simulink model "fuzzyPD_Quadrotor"  (R2025a)
settings: Solver=VariableStepAuto  StartTime=0.0  StopTime=50  RelTol=1e-3
libraries: fuzblock x6, slpidlib x3, uavutilslib x1
settings Model: SimulationMode=accelerator  Creator=vinh1  LastModifiedBy=vinh1
settings RTWCC: Toolchain=MinGW64 | gmake (64-bit Windows)

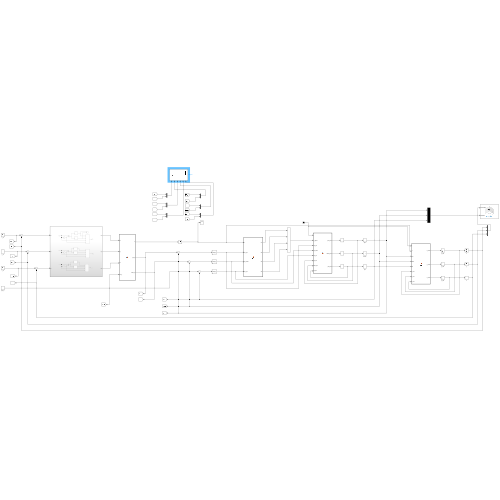
[thumbnail: Simulink's stored preview of the top-level diagram]
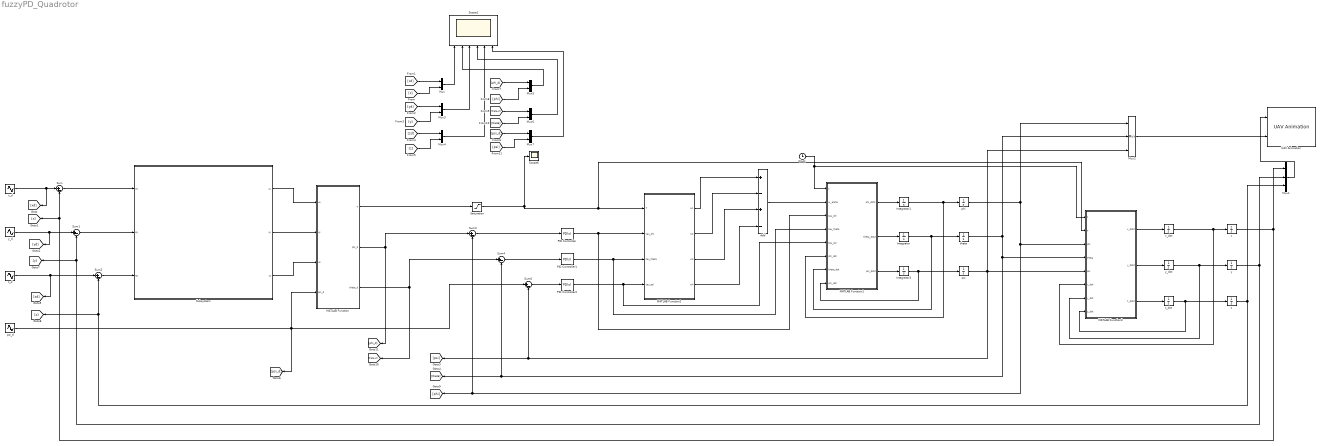
== system fuzzyPD_Quadrotor ==
  Add : Sum  Inputs=+-+-
  Clock : Clock
      settings: Decimation=200
  Integrator : Integrator
  Integrator1 : Integrator
  Integrator3 : Integrator
  MATLAB Function : MATLAB Function  TreatAsAtomicUnit=on
  MATLAB Function1 : MATLAB Function  TreatAsAtomicUnit=on
  MATLAB Function2 : MATLAB Function  TreatAsAtomicUnit=on
  MATLAB Function3 : MATLAB Function  TreatAsAtomicUnit=on
  Mux{,3..7} (6 alike) : Mux  Inputs=2
  Mux1 : Mux  Inputs=3
  Mux2 : Mux  Inputs=3
  PID Controller : slpidlib/PID Controller  Controller=PD  Form=Parallel  TimeDomain=Continuous-time  UseExternalTs=off  SampleTime=-1  IntegratorMethod=Forward Euler  FilterMethod=Forward Euler  ControllerParametersSource=internal  P=0.1  I=1  UseKiTs=off  D=1/3  UseExternalDerivativeSource=off  N=100  UseFilter=on  TunerSelectOption=Transfer Function Based (PID Tuner App)  InitialConditionSource=internal  InitialConditionForIntegrator=0  InitialConditionForFilter=0  DifferentiatorICPrevScaledInput=0  ExternalReset=none  TrackingMode=off  Kt=1  LimitOutput=off  SatLimitsSource=internal  UpperSaturationLimit=inf  LowerSaturationLimit=-inf  LinearizeAsGain=on  AntiWindupMode=none  Kb=1  LimitIntegrator=off  UpperIntegratorSaturationLimit=inf  LowerIntegratorSaturationLimit=-inf  POutMin=[]  POutMax=[]  IOutMin=[]  IOutMax=[]  DOutMin=[]  DOutMax=[]  NOutMin=[]  NOutMax=[]  SumOutMin=[]  SumOutMax=[]  SaturationOutMin=[]  SaturationOutMax=[]  PParamMin=[]  PParamMax=[]  IParamMin=[]  IParamMax=[]  DParamMin=[]  DParamMax=[]  NParamMin=[]  NParamMax=[]  KbParamMin=[]  KbParamMax=[]  KtParamMin=[]  KtParamMax=[]  KbOutMin=[]  KbOutMax=[]  KtOutMin=[]  KtOutMax=[]  IntegratorOutMin=[]  IntegratorOutMax=[]  FilterOutMin=[]  FilterOutMax=[]  SumI1OutMin=[]  SumI1OutMax=[]  SumI2OutMin=[]  SumI2OutMax=[]  SumI3OutMin=[]  SumI3OutMax=[]  SumI4OutMin=[]  SumI4OutMax=[]  SumDOutMin=[]  SumDOutMax=[]  DifferentiatorOutMin=[]  DifferentiatorOutMax=[]  FilterDiffOutCoefMin=[]  FilterDiffOutCoefMax=[]  ReciprocalOutMin=[]  ReciprocalOutMax=[]  SumDenOutMin=[]  SumDenOutMax=[]  SumNumOutMin=[]  SumNumOutMax=[]  DivideOutMin=[]  DivideOutMax=[]  UdiffTsProdOutMin=[]  UdiffTsProdOutMax=[]  NTsProdOutMin=[]  NTsProdOutMax=[]  UintegralTsProdOutMin=[]  UintegralTsProdOutMax=[]  UngainTsProdOutMin=[]  UngainTsProdOutMax=[]  ClampingZeroOutDataTypeStr=Inherit: Inherit via back propagation  ClampingZeroOutMin=[]  ClampingZeroOutMax=[]  FilterDenConstantOutDataTypeStr=Inherit: Inherit via back propagation  FilterDenConstantOutMin=[]  FilterDenConstantOutMax=[]  PCopyOutDataTypeStr=Inherit: Inherit via back propagation  PCopyOutMin=[]  PCopyOutMax=[]  NCopyOutDataTypeStr=Inherit: Inherit via back propagation  NCopyOutMin=[]  NCopyOutMax=[]  IntegratorContinuousStateAttributes=''  IntegratorStateMustResolveToSignalObject=off  IntegratorRTWStateStorageClass=Auto  FilterContinuousStateAttributes=''  FilterStateMustResolveToSignalObject=off  FilterRTWStateStorageClass=Auto  ParallelPVariant=InternalParameters  IdealPVariant=Disabled  IVariant=Disabled  DVariant=InternalParameters  IntegratorVariant=Disabled  SatVariant=Disabled  AWVariant=Disabled  PCopyVariant=Disabled  TRVariant=Disabled  FdbkBlocksVariant=Forward  IdealPFdbkVariant=Disabled  SatFdbkVariant=Disabled  DerivativeFilterVariant=ContFilter  NVariant=InternalParameters  NCopyVariant=Disabled  FilterICVariant=InternalICsFilter  IntegratorICVariant=Disabled  ExternalResetVariant=Disabled  TRSumVariant=Passthrough  SumFdbkVariant=Disabled  SumVariant=Sum_PD  TsampFilterVariant=InternalTs  TsampNgainVariant=Passthrough  TsampIntegralVariant=Disabled_SignalSpec  ExternalSaturationOutDataTypeStr=Inherit: Same as second input  DerivativeSourceVariant=ErrorSignal  PreIntVariant=InternalPreInt
  PID Controller1 : slpidlib/PID Controller  Controller=PD  Form=Parallel  TimeDomain=Continuous-time  UseExternalTs=off  SampleTime=-1  IntegratorMethod=Forward Euler  FilterMethod=Forward Euler  ControllerParametersSource=internal  P=0.1  I=1  UseKiTs=off  D=1/3  UseExternalDerivativeSource=off  N=100  UseFilter=on  TunerSelectOption=Transfer Function Based (PID Tuner App)  InitialConditionSource=internal  InitialConditionForIntegrator=0  InitialConditionForFilter=0  DifferentiatorICPrevScaledInput=0  ExternalReset=none  TrackingMode=off  Kt=1  LimitOutput=off  SatLimitsSource=internal  UpperSaturationLimit=inf  LowerSaturationLimit=-inf  LinearizeAsGain=on  AntiWindupMode=none  Kb=1  LimitIntegrator=off  UpperIntegratorSaturationLimit=inf  LowerIntegratorSaturationLimit=-inf  POutMin=[]  POutMax=[]  IOutMin=[]  IOutMax=[]  DOutMin=[]  DOutMax=[]  NOutMin=[]  NOutMax=[]  SumOutMin=[]  SumOutMax=[]  SaturationOutMin=[]  SaturationOutMax=[]  PParamMin=[]  PParamMax=[]  IParamMin=[]  IParamMax=[]  DParamMin=[]  DParamMax=[]  NParamMin=[]  NParamMax=[]  KbParamMin=[]  KbParamMax=[]  KtParamMin=[]  KtParamMax=[]  KbOutMin=[]  KbOutMax=[]  KtOutMin=[]  KtOutMax=[]  IntegratorOutMin=[]  IntegratorOutMax=[]  FilterOutMin=[]  FilterOutMax=[]  SumI1OutMin=[]  SumI1OutMax=[]  SumI2OutMin=[]  SumI2OutMax=[]  SumI3OutMin=[]  SumI3OutMax=[]  SumI4OutMin=[]  SumI4OutMax=[]  SumDOutMin=[]  SumDOutMax=[]  DifferentiatorOutMin=[]  DifferentiatorOutMax=[]  FilterDiffOutCoefMin=[]  FilterDiffOutCoefMax=[]  ReciprocalOutMin=[]  ReciprocalOutMax=[]  SumDenOutMin=[]  SumDenOutMax=[]  SumNumOutMin=[]  SumNumOutMax=[]  DivideOutMin=[]  DivideOutMax=[]  UdiffTsProdOutMin=[]  UdiffTsProdOutMax=[]  NTsProdOutMin=[]  NTsProdOutMax=[]  UintegralTsProdOutMin=[]  UintegralTsProdOutMax=[]  UngainTsProdOutMin=[]  UngainTsProdOutMax=[]  ClampingZeroOutDataTypeStr=Inherit: Inherit via back propagation  ClampingZeroOutMin=[]  ClampingZeroOutMax=[]  FilterDenConstantOutDataTypeStr=Inherit: Inherit via back propagation  FilterDenConstantOutMin=[]  FilterDenConstantOutMax=[]  PCopyOutDataTypeStr=Inherit: Inherit via back propagation  PCopyOutMin=[]  PCopyOutMax=[]  NCopyOutDataTypeStr=Inherit: Inherit via back propagation  NCopyOutMin=[]  NCopyOutMax=[]  IntegratorContinuousStateAttributes=''  IntegratorStateMustResolveToSignalObject=off  IntegratorRTWStateStorageClass=Auto  FilterContinuousStateAttributes=''  FilterStateMustResolveToSignalObject=off  FilterRTWStateStorageClass=Auto  ParallelPVariant=InternalParameters  IdealPVariant=Disabled  IVariant=Disabled  DVariant=InternalParameters  IntegratorVariant=Disabled  SatVariant=Disabled  AWVariant=Disabled  PCopyVariant=Disabled  TRVariant=Disabled  FdbkBlocksVariant=Forward  IdealPFdbkVariant=Disabled  SatFdbkVariant=Disabled  DerivativeFilterVariant=ContFilter  NVariant=InternalParameters  NCopyVariant=Disabled  FilterICVariant=InternalICsFilter  IntegratorICVariant=Disabled  ExternalResetVariant=Disabled  TRSumVariant=Passthrough  SumFdbkVariant=Disabled  SumVariant=Sum_PD  TsampFilterVariant=InternalTs  TsampNgainVariant=Passthrough  TsampIntegralVariant=Disabled_SignalSpec  ExternalSaturationOutDataTypeStr=Inherit: Same as second input  DerivativeSourceVariant=ErrorSignal  PreIntVariant=InternalPreInt
  PID Controller2 : slpidlib/PID Controller  Controller=PD  Form=Parallel  TimeDomain=Continuous-time  UseExternalTs=off  SampleTime=-1  IntegratorMethod=Forward Euler  FilterMethod=Forward Euler  ControllerParametersSource=internal  P=0.1  I=1  UseKiTs=off  D=1/3  UseExternalDerivativeSource=off  N=100  UseFilter=on  TunerSelectOption=Transfer Function Based (PID Tuner App)  InitialConditionSource=internal  InitialConditionForIntegrator=0  InitialConditionForFilter=0  DifferentiatorICPrevScaledInput=0  ExternalReset=none  TrackingMode=off  Kt=1  LimitOutput=off  SatLimitsSource=internal  UpperSaturationLimit=inf  LowerSaturationLimit=-inf  LinearizeAsGain=on  AntiWindupMode=none  Kb=1  LimitIntegrator=off  UpperIntegratorSaturationLimit=inf  LowerIntegratorSaturationLimit=-inf  POutMin=[]  POutMax=[]  IOutMin=[]  IOutMax=[]  DOutMin=[]  DOutMax=[]  NOutMin=[]  NOutMax=[]  SumOutMin=[]  SumOutMax=[]  SaturationOutMin=[]  SaturationOutMax=[]  PParamMin=[]  PParamMax=[]  IParamMin=[]  IParamMax=[]  DParamMin=[]  DParamMax=[]  NParamMin=[]  NParamMax=[]  KbParamMin=[]  KbParamMax=[]  KtParamMin=[]  KtParamMax=[]  KbOutMin=[]  KbOutMax=[]  KtOutMin=[]  KtOutMax=[]  IntegratorOutMin=[]  IntegratorOutMax=[]  FilterOutMin=[]  FilterOutMax=[]  SumI1OutMin=[]  SumI1OutMax=[]  SumI2OutMin=[]  SumI2OutMax=[]  SumI3OutMin=[]  SumI3OutMax=[]  SumI4OutMin=[]  SumI4OutMax=[]  SumDOutMin=[]  SumDOutMax=[]  DifferentiatorOutMin=[]  DifferentiatorOutMax=[]  FilterDiffOutCoefMin=[]  FilterDiffOutCoefMax=[]  ReciprocalOutMin=[]  ReciprocalOutMax=[]  SumDenOutMin=[]  SumDenOutMax=[]  SumNumOutMin=[]  SumNumOutMax=[]  DivideOutMin=[]  DivideOutMax=[]  UdiffTsProdOutMin=[]  UdiffTsProdOutMax=[]  NTsProdOutMin=[]  NTsProdOutMax=[]  UintegralTsProdOutMin=[]  UintegralTsProdOutMax=[]  UngainTsProdOutMin=[]  UngainTsProdOutMax=[]  ClampingZeroOutDataTypeStr=Inherit: Inherit via back propagation  ClampingZeroOutMin=[]  ClampingZeroOutMax=[]  FilterDenConstantOutDataTypeStr=Inherit: Inherit via back propagation  FilterDenConstantOutMin=[]  FilterDenConstantOutMax=[]  PCopyOutDataTypeStr=Inherit: Inherit via back propagation  PCopyOutMin=[]  PCopyOutMax=[]  NCopyOutDataTypeStr=Inherit: Inherit via back propagation  NCopyOutMin=[]  NCopyOutMax=[]  IntegratorContinuousStateAttributes=''  IntegratorStateMustResolveToSignalObject=off  IntegratorRTWStateStorageClass=Auto  FilterContinuousStateAttributes=''  FilterStateMustResolveToSignalObject=off  FilterRTWStateStorageClass=Auto  ParallelPVariant=InternalParameters  IdealPVariant=Disabled  IVariant=Disabled  DVariant=InternalParameters  IntegratorVariant=Disabled  SatVariant=Disabled  AWVariant=Disabled  PCopyVariant=Disabled  TRVariant=Disabled  FdbkBlocksVariant=Forward  IdealPFdbkVariant=Disabled  SatFdbkVariant=Disabled  DerivativeFilterVariant=ContFilter  NVariant=InternalParameters  NCopyVariant=Disabled  FilterICVariant=InternalICsFilter  IntegratorICVariant=Disabled  ExternalResetVariant=Disabled  TRSumVariant=Passthrough  SumFdbkVariant=Disabled  SumVariant=Sum_PD  TsampFilterVariant=InternalTs  TsampNgainVariant=Passthrough  TsampIntegralVariant=Disabled_SignalSpec  ExternalSaturationOutDataTypeStr=Inherit: Same as second input  DerivativeSourceVariant=ErrorSignal  PreIntVariant=InternalPreInt
  Saturation : Saturate  UpperLimit=130  LowerLimit=0
  Scope1 : Scope  NumInputPorts=6
      settings: ActiveDisplayYMinimum=-0.63879250975812629  ActiveDisplayYMaximum=0.70191029435128827
  Scope6 : Scope
      settings: ActiveDisplayYMinimum=9.3887609139201285  ActiveDisplayYMaximum=11.61040929343401  DataLoggingVariableName=ScopeData6
  Subsystem : Subsystem
  Sum{,1..4,6} (6 alike) : Sum  Inputs=|+-
  UAV Animation : uavutilslib/UAV Animation  NumUAV=1  DynamicUAVConfig=off  UAVType=Multirotor  UAVSize=1  UAVColor=[1 0 0]  UAVTrajectoryAlpha=1  InertialZDirection=Down  RotationFormat=Euler ZYX  DrawMarkers=off  SampleTime=-1
  phi : Integrator
  psi : Integrator
  psi_d : Sin  Amplitude=0  Frequency=pi/10  Phase=pi/2  SampleTime=0
  theta : Integrator  LimitOutput=on  UpperSaturationLimit=85  LowerSaturationLimit=-85
  x : Integrator
  x_d : Sin  Amplitude=0.5  Frequency=pi/20  Phase=pi/2  SampleTime=0
  x_dot : Integrator
  y : Integrator
  y_d : Sin  Amplitude=0.5  Frequency=pi/20  SampleTime=0
  y_dot : Integrator
  z : Integrator  InitialCondition=2  LimitOutput=on  UpperSaturationLimit=100  LowerSaturationLimit=0
  z_d : Sin  Amplitude=0.5  Bias=2  Frequency=pi/20  Phase=3*pi/2  SampleTime=0
  z_dot : Integrator
  wires:
  [zd] -> Mux4/1
  y_d/1 -> Sum1/1, [yd]
  MATLAB Function1/3(psi_dot2) -> Integrator3/1
  [yd] -> Mux3/1
  [phi_d] -> Mux5/1
  MATLAB Function/3(theta_d) -> [theta_d], Sum4/1
  Integrator3/1 -> MATLAB Function1/8(psi_dot), psi/1
  x_dot/1 -> x/1, MATLAB Function3/6(x_dot)
  psi_d/1 -> [psi_d], MATLAB Function/4(psi_d), Sum6/1
  x/1 -> [x], Sum/2, Mux1/1
  [y] -> Mux3/2
  MATLAB Function2/2(w2) -> Add/2
  [theta_d] -> Mux6/1
  MATLAB Function3/2(y_dot2) -> y_dot/1
  MATLAB Function/2(phi_d) -> [phi_d], Sum3/1
  Clock/1 -> MATLAB Function3/1(t), MATLAB Function1/1(t)
  z_d/1 -> [zd], Sum2/1
  Integrator/1 -> theta/1, MATLAB Function1/7(theta_dot)
  z_dot/1 -> z/1, MATLAB Function3/8(z_dot)
  MATLAB Function/1(T) -> Saturation/1
  MATLAB Function3/1(x_dot2) -> x_dot/1
  MATLAB Function2/1(w1) -> Add/1
  z/1 -> Mux1/3, [z], Sum2/2
  Saturation/1 -> MATLAB Function3/2(T), MATLAB Function2/1(T), Scope6/1
  y_dot/1 -> y/1, MATLAB Function3/7(y_dot)
  x_d/1 -> [xd], Sum/1
  MATLAB Function2/4(w4) -> Add/4
  MATLAB Function1/1(phi_dot2) -> Integrator1/1
  MATLAB Function2/3(w3) -> Add/3
  [z] -> Mux4/2
  [phi] -> Mux5/2
  phi/1 -> Mux2/1, Sum3/2, [phi], MATLAB Function3/3(phi)
  Integrator1/1 -> phi/1, MATLAB Function1/6(phi_dot)
  Mux2/1 -> UAV Animation/2
  PID Controller/1 -> MATLAB Function1/3(tau_phi), MATLAB Function2/2(tau_phi)
  Add/1 -> MATLAB Function1/2(w_alpha)
  psi/1 -> MATLAB Function3/5(psi), Mux2/3, [psi], Sum6/2
  [theta] -> Mux6/2
  [psi_d] -> Mux7/1
  MATLAB Function1/2(theta_dot2) -> Integrator/1
  Mux1/1 -> UAV Animation/1
  [psi] -> Mux7/2
  MATLAB Function3/3(z_dot2) -> z_dot/1
  y/1 -> Mux1/2, Sum1/2, [y]
  theta/1 -> Mux2/2, MATLAB Function3/4(theta), Sum4/2, [theta]
  PID Controller1/1 -> MATLAB Function2/3(tau_theta), MATLAB Function1/4(tau_theta)
  Sum6/1 -> PID Controller2/1
  PID Controller2/1 -> MATLAB Function2/4(tau_psi), MATLAB Function1/5(tau_psi)
  Sum3/1 -> PID Controller/1
  Sum4/1 -> PID Controller1/1
  Subsystem/1(ux) -> MATLAB Function/1(ux)
  Subsystem/2(uy) -> MATLAB Function/2(uy)
  Subsystem/3(uz) -> MATLAB Function/3(uz)
  Sum2/1 -> Subsystem/3(ez)
  Sum1/1 -> Subsystem/2(ey)
  Sum/1 -> Subsystem/1(ex)
  Mux5/1 -> Scope1/2
  Mux3/1 -> Scope1/3
  Mux4/1 -> Scope1/5
  Mux6/1 -> Scope1/4
  Mux7/1 -> Scope1/6
  [x] -> Mux/2
  [xd] -> Mux/1
  Mux/1 -> Scope1/1

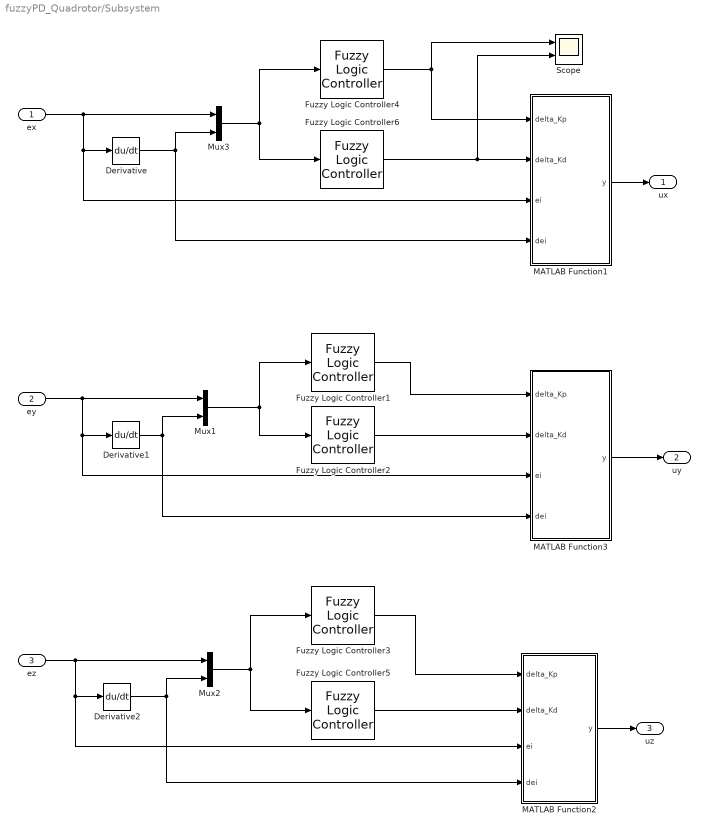
== system fuzzyPD_Quadrotor/Subsystem ==
  ex : Inport
  ey : Inport  Port=2
  ez : Inport  Port=3
  Derivative : Derivative
  Derivative1 : Derivative
  Derivative2 : Derivative
  Fuzzy Logic Controller1 : fuzblock/Fuzzy Logic  Controller  FIS='delKp.fis'  OutputSampleNumber=101  DataType=double  UseLookupTable=off  NumBreakpoints=10  FuzzifiedInputs=off  RuleFiringStrengths=off  RuleOutputs=off  AggregatedOutputs=off  SimulateUsing=Interpreted execution  OutOfRangeInputValueMessage=warning  NoRuleFiredMessage=warning  EmptyOutputFuzzySetMessage=warning
  Fuzzy Logic Controller2 : fuzblock/Fuzzy Logic  Controller  FIS='delKd.fis'  OutputSampleNumber=101  DataType=double  UseLookupTable=on  NumBreakpoints=10  FuzzifiedInputs=off  RuleFiringStrengths=off  RuleOutputs=off  AggregatedOutputs=off  SimulateUsing=Interpreted execution  OutOfRangeInputValueMessage=warning  NoRuleFiredMessage=warning  EmptyOutputFuzzySetMessage=warning
  Fuzzy Logic Controller3 : fuzblock/Fuzzy Logic  Controller  FIS='delKp.fis'  OutputSampleNumber=101  DataType=double  UseLookupTable=off  NumBreakpoints=10  FuzzifiedInputs=off  RuleFiringStrengths=off  RuleOutputs=off  AggregatedOutputs=off  SimulateUsing=Interpreted execution  OutOfRangeInputValueMessage=warning  NoRuleFiredMessage=warning  EmptyOutputFuzzySetMessage=warning
  Fuzzy Logic Controller4 : fuzblock/Fuzzy Logic  Controller  FIS='delKp.fis'  OutputSampleNumber=101  DataType=double  UseLookupTable=off  NumBreakpoints=10  FuzzifiedInputs=off  RuleFiringStrengths=off  RuleOutputs=off  AggregatedOutputs=off  SimulateUsing=Interpreted execution  OutOfRangeInputValueMessage=warning  NoRuleFiredMessage=warning  EmptyOutputFuzzySetMessage=warning
  Fuzzy Logic Controller5 : fuzblock/Fuzzy Logic  Controller  FIS='delKd.fis'  OutputSampleNumber=101  DataType=double  UseLookupTable=on  NumBreakpoints=10  FuzzifiedInputs=off  RuleFiringStrengths=off  RuleOutputs=off  AggregatedOutputs=off  SimulateUsing=Interpreted execution  OutOfRangeInputValueMessage=warning  NoRuleFiredMessage=warning  EmptyOutputFuzzySetMessage=warning
  Fuzzy Logic Controller6 : fuzblock/Fuzzy Logic  Controller  FIS='delKd.fis'  OutputSampleNumber=101  DataType=double  UseLookupTable=on  NumBreakpoints=10  FuzzifiedInputs=off  RuleFiringStrengths=off  RuleOutputs=off  AggregatedOutputs=off  SimulateUsing=Interpreted execution  OutOfRangeInputValueMessage=warning  NoRuleFiredMessage=warning  EmptyOutputFuzzySetMessage=warning
  MATLAB Function1 : MATLAB Function  TreatAsAtomicUnit=on
  MATLAB Function2 : MATLAB Function  TreatAsAtomicUnit=on
  MATLAB Function3 : MATLAB Function  TreatAsAtomicUnit=on
  Mux1 : Mux  Inputs=2
  Mux2 : Mux  Inputs=2
  Mux3 : Mux  Inputs=2
  Scope : Scope  NumInputPorts=2
      settings: ActiveDisplayYMinimum=1.0209922135139156  ActiveDisplayYMaximum=2.7064980431565342  DataLoggingVariableName=ScopeData7
  ux : Outport
  uy : Outport  Port=2
  uz : Outport  Port=3
  wires:
  Derivative2/1 -> MATLAB Function2/4(dei), Mux2/2
  Mux2/1 -> Fuzzy Logic Controller5/1, Fuzzy Logic Controller3/1
  MATLAB Function3/1(y) -> uy/1
  MATLAB Function2/1(y) -> uz/1
  Derivative1/1 -> MATLAB Function3/4(dei), Mux1/2
  Mux1/1 -> Fuzzy Logic Controller2/1, Fuzzy Logic Controller1/1
  Derivative/1 -> MATLAB Function1/4(dei), Mux3/2
  MATLAB Function1/1(y) -> ux/1
  Mux3/1 -> Fuzzy Logic Controller6/1, Fuzzy Logic Controller4/1
  Fuzzy Logic Controller6/1 -> MATLAB Function1/2(delta_Kd), Scope/2
  Fuzzy Logic Controller4/1 -> MATLAB Function1/1(delta_Kp), Scope/1
  Fuzzy Logic Controller1/1 -> MATLAB Function3/1(delta_Kp)
  Fuzzy Logic Controller2/1 -> MATLAB Function3/2(delta_Kd)
  Fuzzy Logic Controller5/1 -> MATLAB Function2/2(delta_Kd)
  Fuzzy Logic Controller3/1 -> MATLAB Function2/1(delta_Kp)
  ez/1 -> MATLAB Function2/3(ei), Derivative2/1, Mux2/1
  ey/1 -> MATLAB Function3/3(ei), Derivative1/1, Mux1/1
  ex/1 -> Mux3/1, MATLAB Function1/3(ei), Derivative/1

== matlab function fuzzyPD_Quadrotor/Subsystem/MATLAB Function2 ==
  data: delta_Kp input; y output; delta_Kd input; ei input; dei input
function y = fcn(delta_Kp, delta_Kd,ei,dei)

y = (0.1 + delta_Kp)*ei + ((1/3) + delta_Kd)*dei ;

== matlab function fuzzyPD_Quadrotor/MATLAB Function1 ==
  data: t input; w_alpha input; phi_dot2 output; tau_phi input; tau_theta input; tau_psi input; theta_dot2 output; psi_dot2 output; phi_dot input; theta_dot input; psi_dot input
function [phi_dot2, theta_dot2, psi_dot2] = fcn(t, w_alpha, tau_phi, tau_theta, tau_psi, phi_dot, theta_dot, psi_dot)


Ixx = 0.01 ;
Iyy = 0.01 ; 
Izz = 0.0148 ;
Ir = 2.83e-5 ;

%dphi = 0.2*sin(2*t) ;
%dtheta = 0.2*sin(2*t) ;
%dpsi = 0.1*sin(t) ;



phi_dot2 = theta_dot*psi_dot*(Iyy - Izz)/Ixx - theta_dot*w_alpha*Ir/Ixx + tau_phi/Ixx; %+ dphi

theta_dot2 = phi_dot*psi_dot*(Izz - Ixx)/Iyy + phi_dot*w_alpha*Ir/Iyy + tau_theta/Iyy %+ dtheta

psi_dot2 = phi_dot*theta_dot*(Ixx - Iyy)/Izz + tau_psi/Ixx; %+ dpsi

end

== matlab function fuzzyPD_Quadrotor/MATLAB Function ==
  data: ux input; T output; uy input; uz input; psi_d input; phi_d output; theta_d output
function [T, phi_d, theta_d] = fcn(ux, uy, uz, psi_d)

m = 1.121 ;
g = 9.81 ;

T = m*sqrt( (ux)^2 + (uy)^2 + (uz + g)^2);

phi_d = asin((ux*sin(psi_d) - uy*cos(psi_d)) / (T/m));

theta_d = atan((ux*cos(psi_d) + uy*sin(psi_d)) / (uz + g));

== matlab function fuzzyPD_Quadrotor/MATLAB Function2 ==
  data: T input; w1 output; tau_phi input; tau_theta input; tau_psi input; w2 output; w3 output; w4 output
function [w1, w2, w3, w4] = fcn(T, tau_phi, tau_theta, tau_psi)

k = 2.98e-5 ;
l = 0.25 ;
b = 3.23e-7 ;

w1 = sqrt(max(0,(T/(4*k)) - (tau_theta/(2*k*l)) - (tau_psi/(4*b))));

w2 = sqrt(max(0,(T/(4*k)) - (tau_phi /(2*k*l)) + (tau_psi/(4*b))));

w3 = sqrt(max(0,(T/(4*k)) + (tau_theta/(2*k*l)) - (tau_psi/(4*b))));

w4 = sqrt(max(0,(T/(4*k)) + (tau_phi /(2*k*l)) + (tau_psi/(4*b))));

end

== matlab function fuzzyPD_Quadrotor/MATLAB Function3 ==
  data: t input; T input; phi input; x_dot2 output; theta input; psi input; x_dot input; y_dot2 output; z_dot2 output; y_dot input; z_dot input
function [x_dot2, y_dot2, z_dot2] = fcn(t, T, phi, theta, psi, x_dot, y_dot, z_dot)



Ax = 5.56e-4 ;
Ay = 5.56e-4 ;
Az = 6.35e-4 ;

m = 1.121 ;
g = 9.81 ;

%dx = 0.3*sin(t) ;
%dy = 0.3*sin(t) ;
%dz = 0.1*sin(0.5*t) ;

x_dot2 = (T/m)*( cos(phi)*sin(theta)*cos(psi) + sin(phi)*sin(psi)) - (Ax/m)*x_dot; %+ dx;

y_dot2 = (T/m)*( cos(phi)*sin(theta)*sin(psi) - sin(phi)*cos(psi)) - (Ay/m)*y_dot; %+ dy;

z_dot2 = (T/m)*cos(phi)*cos(theta) - g - (Az/m)*z_dot;% + dz;

end

== matlab function fuzzyPD_Quadrotor/Subsystem/MATLAB Function1 ==
  data: delta_Kp input; y output; delta_Kd input; ei input; dei input
function y = fcn(delta_Kp, delta_Kd,ei,dei)

y = (0.1 + delta_Kp)*ei + ((1/3) + delta_Kd)*dei ;

== matlab function fuzzyPD_Quadrotor/Subsystem/MATLAB Function3 ==
  data: delta_Kp input; y output; delta_Kd input; ei input; dei input
function y = fcn(delta_Kp, delta_Kd,ei,dei)

y = (0.1 + delta_Kp)*ei + ((1/3) + delta_Kd)*dei ;
